simulink model "ex23_simulink"  (R2021b)
settings: Solver=VariableStepAuto  StartTime=0.0  StopTime=100.0  RelTol=1e-3
values from neighbouring files (symbols this model uses):
  D = [ 1,2,4]    [ex10.m]    (also in ex22.m = 0.4; ex23.m = 0.1; ex34.m = [C(2) C(4);d1 0])
  J = JM +JL    (= 1.1)    [ex23.m]
  Kg = 0.1    [ex23.m]
  KM = 1    [ex23.m]
  L = 1e-3    (= 0.001)    [ex10.m]    (also in ex23.m = 0.2; ex27.m = 0.0001; ex27c.m = 0.0001; ex8.m)
  R = Rv(n)    [ex10.m]    (also in ex22.m = 0.2; ex23.m = 1.3; ex27c.m = 2.8; ex8.m = 10)
  TL = 5    [ex23.m]
settings Model: Creator=rafam  LastModifiedBy=rafam

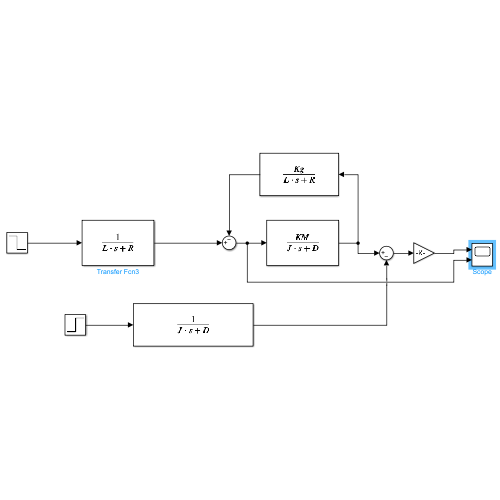
[thumbnail: Simulink's stored preview of the top-level diagram]
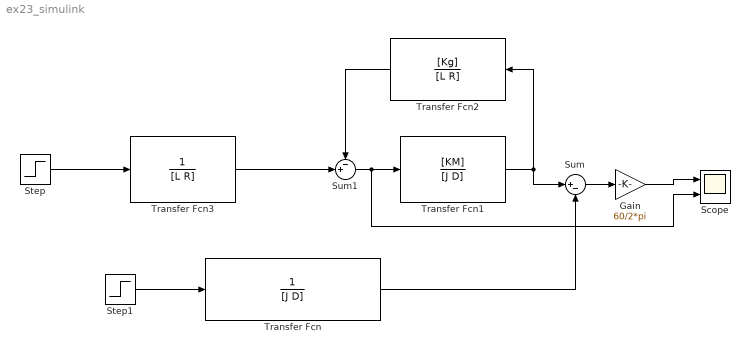
== system ex23_simulink ==
  Gain : Gain  Gain=60/2*pi
  Scope : Scope  NumInputPorts=2
  Step : Step  Time=0  Before=10  SampleTime=0
  Step1 : Step  Time=50  After=TL  SampleTime=0
  Sum : Sum  Inputs=|+-
  Sum1 : Sum  Inputs=-+|
  Transfer Fcn : TransferFcn  Denominator=[J D]
  Transfer Fcn1 : TransferFcn  Numerator=[KM]  Denominator=[J D]
  Transfer Fcn2 : TransferFcn  Numerator=[Kg]  Denominator=[L R]
  Transfer Fcn3 : TransferFcn  Denominator=[L R]
  wires:
  Step/1 -> Transfer Fcn3/1
  Step1/1 -> Transfer Fcn/1
  Sum1/1 -> Scope/2, Transfer Fcn1/1
  Sum/1 -> Gain/1
  Transfer Fcn1/1 -> Sum/1, Transfer Fcn2/1
  Transfer Fcn3/1 -> Sum1/2
  Transfer Fcn2/1 -> Sum1/1
  Transfer Fcn/1 -> Sum/2
  Gain/1 -> Scope/1
